simulink model "vehicle_SSC"  (R2022b)
settings: Solver=VariableStepAuto  StartTime=0.0  StopTime=10.0  RelTol=1e-3
PreLoadFcn:
  | vehicleObject = vehicle.ParallelSUV;
libraries: sdl_lib x2, nesl_utility x1
settings Model: Creator=grouleau  LastModifiedBy=GeraldoFranciscodeSo
settings ModelReferenceCC: EnableRefExpFcnMdlSchedulingChecks=on

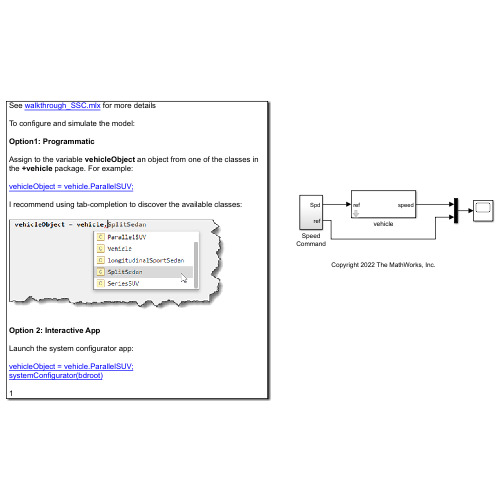
[thumbnail: Simulink's stored preview of the top-level diagram]
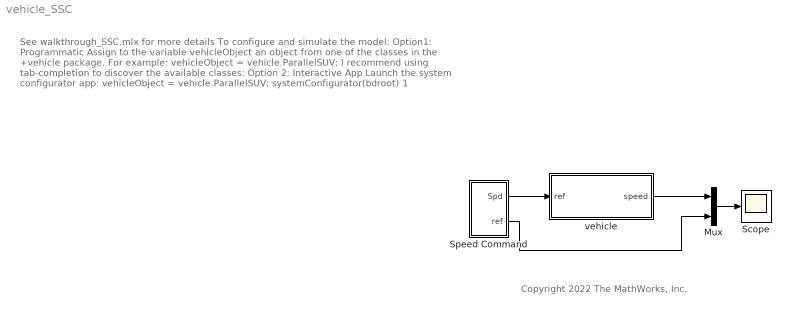
== system vehicle_SSC ==
  note: See walkthrough_SSC.mlx for more details
      |
      | To configure and simulate the model:
      |
      | Option1: Programmatic
      |
      | Assign to the variable vehicleObject an object from one of the classes in the +vehicle package. For example:
      |
      | vehicleObject = vehicle.ParallelSUV;
      |
      | I recommend using tab-completion to discover the available classes:
      |
      | Option 2: Interactive App
      |
      | Launch the system configurator app:
      |
      | vehicleObject = vehicle.ParallelSUV;
      | systemConfigurator(bdroot)
      |
      | 1
  note: Copyright 2022 The MathWorks, Inc.
  Mux : Mux  Inputs=2
  Scope : Scope
  Speed Command : Subsystem
  vehicle : Subsystem  mask(slPart){obj=vehicleObject}
      mask prompts: obj "slPart Object:"
      mask help: This subsystem implements a simplified vehicle with multiple hybrid drivetrain and parameterizations. To configure the vehicle, assign an object instantiated from one of the class in the "+vehicle" folder.
      mask init:
      | obj.maskInit(gcb);
      mask DialogControl Control2 Prompt: See walkthrough_SSC.mlx for more examples
      mask DialogControl Control2 Callback: open('walkthrough_SSC.mlx')
      mask DialogControl Container3 Prompt: Example
      mask DialogControl Control3 Prompt: vehicleObject = vehicle.ParallelSUV;
      mask DialogControl Control3 Callback: vehicleObject = vehicle.ParallelSUV;
  wires:
  Speed Command/1(Spd) -> vehicle/1(ref)
  Mux/1 -> Scope/1
  vehicle/1(speed) -> Mux/1
  Speed Command/2(ref) -> Mux/2

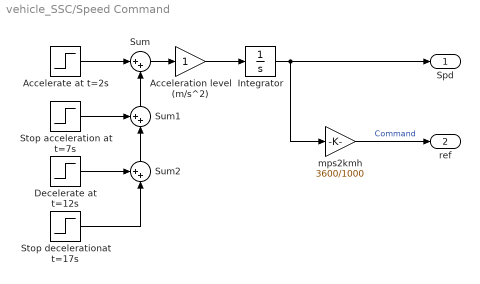
== system vehicle_SSC/Speed Command ==
  Accelerate at t=2s : Step  Time=2  SampleTime=0
  Acceleration level (m/s^2) : Gain
  Decelerate at t=12s : Step  Time=12  After=-1  SampleTime=0
  Integrator : Integrator  InitialCondition=15
  Stop acceleration at t=7s : Step  Time=7  After=-1  SampleTime=0
  Stop decelerationat t=17s : Step  Time=17  SampleTime=0
  Sum : Sum  Inputs=|++
  Sum1 : Sum  Inputs=++|
  Sum2 : Sum  Inputs=++|
  mps2kmh : Gain  Gain=3600/1000
  Spd : Outport  VectorParamsAs1DForOutWhenUnconnected=off
  ref : Outport  Port=2  VectorParamsAs1DForOutWhenUnconnected=off
  wires:
  Integrator/1 -> mps2kmh/1, Spd/1
  mps2kmh/1 -> ref/1  "Command"
  Stop decelerationat t=17s/1 -> Sum2/2
  Decelerate at t=12s/1 -> Sum2/1
  Acceleration level (m/s^2)/1 -> Integrator/1
  Sum2/1 -> Sum1/2
  Sum1/1 -> Sum/2
  Stop acceleration at t=7s/1 -> Sum1/1
  Sum/1 -> Acceleration level (m/s^2)/1
  Accelerate at t=2s/1 -> Sum/1

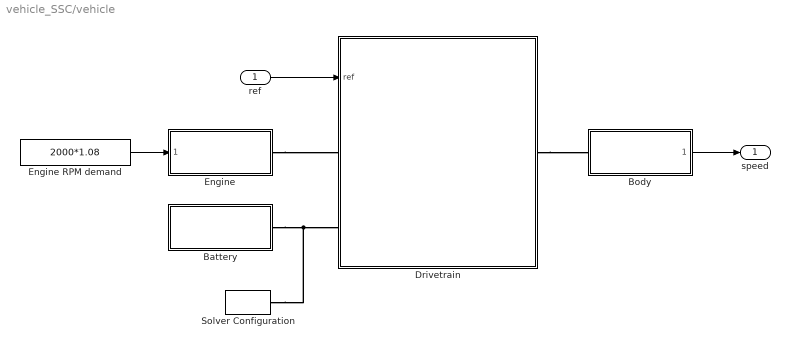
== system vehicle_SSC/vehicle ==
  ref : Inport
  Battery : Subsystem  ReferencedSubsystem=battery_ss  obj=obj.Battery
  Body : Subsystem  ReferencedSubsystem=body_ss  obj=obj.Body
  Drivetrain : Subsystem  Variant=on  VariantControlMode=label  LabelModeActiveChoice=drivetrain.Split  mask(slPart){obj=obj.Drivetrain}
      mask prompts: obj "slPart Object:"
      mask help: Container block for all slPart blocks
      mask init:
      | obj.maskInit(gcb);
  Engine : Subsystem  ReferencedSubsystem=engine_ss  obj=obj.Engine
  Engine RPM demand : Constant  Value=2000*1.08
  Solver Configuration : nesl_utility/Solver Configuration  PhysicalDomain=network_engine_domain  SubClassName=solver  LeftPortType=input  RightPortType=generic  Tones=[]  Harmonics=[]  SimulateNoise=off  Profile=off  UseLocalSampling=off  EnableSwitchedLinearOptims=on  FrequencyDomain=off  UseCCode=off  RelTol=0.001  AbsTol=1e-06  MinStep=1e-09  ToWorkspace=off  RevertToSquareIcSolve=off  NumHomotopyIterations=100  PhasorMode=off  PhasorModeNumHarmonics=1  ConsistencySolver=NEWTON_FTOL  IndexReductionMethod=DerivativeReplacement  DoDC=off  ResidualTolerance=1e-9  ConsistencyTolSource=GLOBAL  ConsistencyAbsTol=0.001  ConsistencyRelTol=0.001  ConsistencyTolFactor=0.001  UseLocalSolver=off  LocalSolverChoice=NE_PARTITIONING_ADVANCER  ResolveIndetEquations=on  FunctionEvalNumThread=1  LocalSolverSampleTime=0.005  DoFixedCost=off  MaxNonlinIter=5  MaxModeIter=2  ComputeImpulses=off  ImpulseIterations=2  LinearAlgebra=auto  LinearAlgebraNumThread=0  EquationFormulation=NE_TIME_EF  DelaysMemoryBudget=1024  AutomaticFiltering=on  FilteringTimeConstant=0.001  PartitionStorageMethod=EXHAUSTIVE  PartitionMemoryBudget=1024  PartitionMethod=ROBUST
  speed : Outport
  wires:
  Body/1 -> speed/1
  ref/1 -> Drivetrain/1(ref)
  Engine RPM demand/1 -> Engine/1
  connections:
  Engine/RConn1 -- Drivetrain/LConn1
  Battery/RConn1 -- Solver Configuration/RConn1 -- Drivetrain/LConn2
  Drivetrain/RConn1 -- Body/LConn1

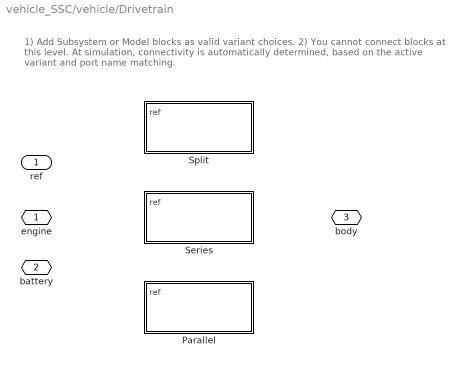
== system vehicle_SSC/vehicle/Drivetrain ==
  note: 1) Add Subsystem or Model blocks as valid variant choices.
      | 2) You cannot connect blocks at this level. At simulation, connectivity is automatically
      | determined, based on the active variant and port name matching.
  ref : Inport
  Parallel : Subsystem  VariantControl=drivetrain.Parallel
  Series : Subsystem  VariantControl=drivetrain.Series
  Split : Subsystem  VariantControl=drivetrain.Split
  engine : PMIOPort  Side=Left
  battery : PMIOPort  Port=2  Side=Left
  body : PMIOPort  Port=3  Side=Right

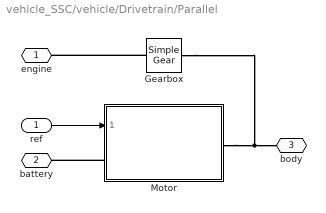
== system vehicle_SSC/vehicle/Drivetrain/Parallel ==
  ref : Inport
  Gearbox : sdl_lib/Gears/Simple Gear  ratio=4.27  rotation_direction=sdl.enum.shaftOutputDirection.same  friction_model=sdl.enum.gear_efficiencies_load.constant  T_noload=0.1 N*m  T_nom=5 N*m  efficiency_nom=0.8  efficiency=0.95  temperature_TLU=[ 280 300 320 ] K  load_TLU=[ 1 5 10 ] N*m  efficiency_TLU=[ 0.95 0.9 0.85 ]  efficiency_TLU2=[ 0.85 0.8 0.75; 0.95 0.9 0.85; 0.85 0.8 0.7 ]  w_thr=0.01 rad/s  pwr_thr=0.001 W  backlash_model=sdl.enum.backlashModel.Off  backlash_distance=1e-3 mm  x0=0 mm  r_base=0.1 m  hardstop_model=simscape.enum.hardstop.smooth  transition=1e-4 mm  backlash_stiffness=1e7 N/m  backlash_damping=1e6 N/(m/s)  e=0  v_tol=0.001 m/s  mu_visc=[ 0 0 ] N*m/(rad/s)  enable_faults=simscape.enum.onoff.off  efficiency_fault=0.05  external_fault=simscape.enum.onoff.off  temporal_fault=simscape.enum.onoff.off  fault_time=5 s  fault_angles=pi / 12 rad  report_fault=simscape.enum.assert.action.none  thermal_mass=50 J/K  temperature_specify=off  temperature_priority=High  temperature=300 K  temperature_nominal_specify=off  temperature_nominal_unit=K  temperature_nominal_value=1  x_backlash_specify=off  x_backlash_priority=None  x_backlash=0 mm  x_backlash_nominal_specify=off  x_backlash_nominal_unit=mm  x_backlash_nominal_value=1  f_hardstop_specify=off  f_hardstop_priority=None  f_hardstop=0 N  f_hardstop_nominal_specify=off  f_hardstop_nominal_unit=N  f_hardstop_nominal_value=1  v_backlash_specify=off  v_backlash_priority=None  v_backlash=0 m/s  v_backlash_nominal_specify=off  v_backlash_nominal_unit=m/s  v_backlash_nominal_value=1
  Motor : Subsystem  ReferencedSubsystem=motor_ss  obj=obj.Motor
  engine : PMIOPort  Side=Left
  battery : PMIOPort  Port=2  Side=Left
  body : PMIOPort  Port=3  Side=Right
  wires:
  ref/1 -> Motor/1
  connections:
  Motor/RConn1 -- Gearbox/RConn1 -- body/RConn1
  Motor/LConn1 -- battery/RConn1
  Gearbox/LConn1 -- engine/RConn1

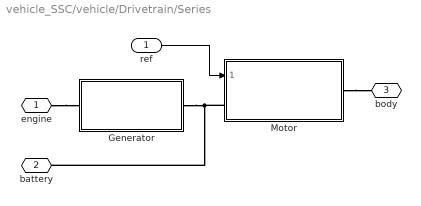
== system vehicle_SSC/vehicle/Drivetrain/Series ==
  ref : Inport
  Generator : Subsystem  ReferencedSubsystem=generator_ss  obj=obj.Generator
  Motor : Subsystem  ReferencedSubsystem=motor_ss  obj=obj.Motor
  engine : PMIOPort  Side=Left
  battery : PMIOPort  Port=2  Side=Left
  body : PMIOPort  Port=3  Side=Right
  wires:
  ref/1 -> Motor/1
  connections:
  engine/RConn1 -- Generator/LConn1
  Generator/RConn1 -- Motor/LConn1 -- battery/RConn1
  Motor/RConn1 -- body/RConn1

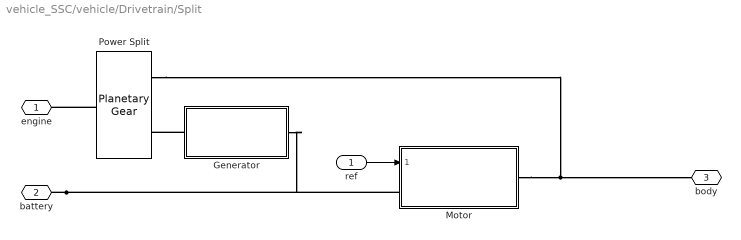
== system vehicle_SSC/vehicle/Drivetrain/Split ==
  ref : Inport
  Generator : Subsystem  ReferencedSubsystem=generator_ss  obj=obj.Generator
  Motor : Subsystem  ReferencedSubsystem=motor_ss  obj=obj.Motor
  Power Split : sdl_lib/Gears/Planetary Gear  rs_ratio=2  friction_model=2  efficiency=[ 0.96 0.98 ]  temperature_TLU=[ 280 300 320 ] K  efficiency_sp_TLU=[ 0.95 0.9 0.85 ]  efficiency_rp_TLU=[ 0.95 0.9 0.85 ]  pwr_thr=[ 0.001 0.001 ] W  mu_visc=[ 0 0 ] N*m/(rad/s)  model_inertia=0  planet_inertia=0.001 kg*m^2  thermal_mass=50 J/K  T_init=300 K
  engine : PMIOPort  Side=Left
  battery : PMIOPort  Port=2  Side=Left
  body : PMIOPort  Port=3  Side=Right
  wires:
  ref/1 -> Motor/1
  connections:
  Power Split/RConn1 -- body/RConn1 -- Motor/RConn1
  battery/RConn1 -- Motor/LConn1 -- Generator/RConn1
  Generator/LConn1 -- Power Split/RConn2
  Power Split/LConn1 -- engine/RConn1
